simulink model "dmpwalk2014"  (R2018b)
settings: Solver=VariableStepAuto  StartTime=0.0  StopTime=100  RelTol=1e-3
values from neighbouring files (symbols this model uses):
  arm_radius = leg_radius    (= 0.01)    [Nao_paramter.m]
  foot_height = 0.02    [Nao_paramter.m]
  foot_length = 0.1    [Nao_paramter.m]
  foot_mass = 0.17184    [Nao_paramter.m]
  foot_width = 0.05    [Nao_paramter.m]
  ground_height = 0.0025    [Nao_paramter.m]
  ground_length = 5    [Nao_paramter.m]
  ground_width = 2    [Nao_paramter.m]
  hand_mass = 0.18533    [Nao_paramter.m]
  head_mass = 0.60533    [Nao_paramter.m]
  hip_mass = 0.14053    [Nao_paramter.m]
  hip_off_Y = 0.05    [Nao_paramter.m]
  hip_off_Z = 0.085    [Nao_paramter.m]
  leg_radius = 0.01    [Nao_paramter.m]
  lowerarm_length = 0.05595    [Nao_paramter.m]
  lowerarm_mass = 0.07761    [Nao_paramter.m]
  neck_length = 0.03    [Nao_paramter.m]
  neck_mass = 0.07842    [Nao_paramter.m]
  neck_off_Z = 0.1265    [Nao_paramter.m]
  shoulder_mass = 0.09304    [Nao_paramter.m]
  thigh_mass = 0.38968    [Nao_paramter.m]
  tibia_mass = 0.30142    [Nao_paramter.m]
  torso_height = foot_height + tibia_length + thigh_length + 0.5*hip_off_Z    (= 0.2654)    [Nao_paramter.m]
  torso_mass = 1.0496    [Nao_paramter.m]
  upperarm_length = 0.105    [Nao_paramter.m]
  upperarm_mass = 0.15777    [Nao_paramter.m]
undefined symbols (not defined in the file or in its folder): sigbuilder_block, X, Y, Z
libraries: sm_lib x87, nesl_utility x15, Contact_Forces_Lib x10
(part 4 of 5)

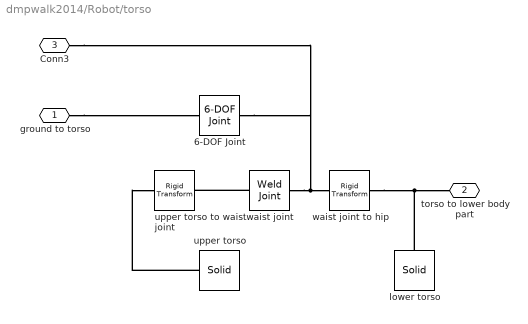
== system dmpwalk2014/Robot/torso ==
  " waist joint" : sm_lib/Joints/Weld Joint  SenseConstraintForce=off  SenseConstraintForceX=off  SenseConstraintForceY=off  SenseConstraintForceZ=off  SenseConstraintTorque=off  SenseConstraintTorqueX=off  SenseConstraintTorqueY=off  SenseConstraintTorqueZ=off  SenseTotalForce=off  SenseTotalForceX=off  SenseTotalForceY=off  SenseTotalForceZ=off  SenseTotalTorque=off  SenseTotalTorqueX=off  SenseTotalTorqueY=off  SenseTotalTorqueZ=off  CompositeWrenchDir=FollowerOnBase  CompositeWrenchFrame=BaseFrame
  6-DOF Joint : sm_lib/Joints/6-DOF Joint  SenseConstraintForce=off  SenseConstraintForceX=off  SenseConstraintForceY=off  SenseConstraintForceZ=off  SenseConstraintTorque=off  SenseConstraintTorqueX=off  SenseConstraintTorqueY=off  SenseConstraintTorqueZ=off  SenseTotalForce=off  SenseTotalForceX=off  SenseTotalForceY=off  SenseTotalForceZ=off  SenseTotalTorque=off  SenseTotalTorqueX=off  SenseTotalTorqueY=off  SenseTotalTorqueZ=off  CompositeWrenchDir=FollowerOnBase  CompositeWrenchFrame=BaseFrame  PxEquilibriumPosition=0  PxEquilibriumPositionUnits=m  PxSpringStiffness=1000  PxSpringStiffnessUnits=N/m  PxDampingCoefficient=800  PxDampingCoefficientUnits=N/(m/s)  PxTorqueActuationMode=NoTorque  PxMotionActuationMode=ComputedMotion  PxSensePosition=off  PxSenseVelocity=off  PxSenseAcceleration=off  PxSenseTorqueForce=off  PxPositionTargetSpecify=on  PxPositionTargetPriority=High  PxPositionTargetValue=0  PxPositionTargetValueUnits=m  PxVelocityTargetSpecify=off  PxVelocityTargetPriority=High  PxVelocityTargetValue=0  PxVelocityTargetValueUnits=m/s  PyEquilibriumPosition=0  PyEquilibriumPositionUnits=m  PySpringStiffness=1000  PySpringStiffnessUnits=N/m  PyDampingCoefficient=800  PyDampingCoefficientUnits=N/(m/s)  PyTorqueActuationMode=NoTorque  PyMotionActuationMode=ComputedMotion  PySensePosition=off  PySenseVelocity=off  PySenseAcceleration=off  PySenseTorqueForce=off  PyPositionTargetSpecify=on  PyPositionTargetPriority=High  PyPositionTargetValue=0  PyPositionTargetValueUnits=m  PyVelocityTargetSpecify=off  PyVelocityTargetPriority=High  PyVelocityTargetValue=0  PyVelocityTargetValueUnits=m/s  PzEquilibriumPosition=0  PzEquilibriumPositionUnits=m  PzSpringStiffness=1000  PzSpringStiffnessUnits=N/m  PzDampingCoefficient=800  PzDampingCoefficientUnits=N/(m/s)  PzTorqueActuationMode=NoTorque  PzMotionActuationMode=ComputedMotion  PzSensePosition=off  PzSenseVelocity=off  PzSenseAcceleration=off  PzSenseTorqueForce=off  PzPositionTargetSpecify=on  PzPositionTargetPriority=High  PzPositionTargetValue=torso_height+0.001  PzPositionTargetValueUnits=m  PzVelocityTargetSpecify=off  PzVelocityTargetPriority=High  PzVelocityTargetValue=0  PzVelocityTargetValueUnits=m/s  SphDefPosRotationMethod=None  SphDefPosRotationAngleUnits=deg  SphDefPosRotationStandardAxis=+Z  SphDefPosRotationAngle=0.0  SphDefPosRotationArbitraryAxis=[0 0 1]  SphDefPosFollAlignAxisA=+X  SphDefPosBaseAlignAxisA=+Y  SphDefPosFollAlignAxisB=+Y  SphDefPosBaseAlignAxisB=+Z  SphDefPosRotationSequenceAxes=FollowerAxes  SphDefPosRotationSequence=XYX  SphDefPosRotationSequenceAngles=[0 0 0]  SphDefPosRotationSequenceAnglesUnits=deg  SphDefPosRotationMatrix=[1 0 0; 0 1 0; 0 0 1]  SphEqPosRotationMethod=None  SphEqPosRotationAngleUnits=deg  SphEqPosRotationStandardAxis=+Z  SphEqPosRotationAngle=0.0  SphEqPosRotationArbitraryAxis=[0 0 1]  SphEqPosFollAlignAxisA=+X  SphEqPosBaseAlignAxisA=+Y  SphEqPosFollAlignAxisB=+Y  SphEqPosBaseAlignAxisB=+Z  SphEqPosRotationSequenceAxes=FollowerAxes  SphEqPosRotationSequence=XYX  SphEqPosRotationSequenceAngles=[0 0 0]  SphEqPosRotationSequenceAnglesUnits=deg  SphEqPosRotationMatrix=[1 0 0; 0 1 0; 0 0 1]  SphSpringStiffness=1000  SphSpringStiffnessUnits=N*m/deg  SphDampingCoefficient=1000  SphDampingCoefficientUnits=N*m/(rad/s)  SphActuateTorqueX=off  SphActuateTorqueY=off  SphActuateTorqueZ=off  SphActuateTorque=off  SphTorqueActuationMode=NoTorque  SphMotionActuationMode=ComputedMotion  SphActuationFrame=BaseFrame  SphSensePosition=off  SphSenseVelocityX=off  SphSenseVelocityY=off  SphSenseVelocityZ=off  SphSenseVelocity=off  SphSenseAccelerationX=off  SphSenseAccelerationY=off  SphSenseAccelerationZ=off  SphSenseAcceleration=off  SphSenseTorqueX=off  SphSenseTorqueY=off  SphSenseTorqueZ=off  SphSenseTorqueForce=off  SphSensingFrame=BaseFrame  SphPositionTargetRotationMethod=None  SphPositionTargetRotationAngleUnits=deg  SphPositionTargetRotationStandardAxis=+Z  SphPositionTargetRotationAngle=0.0  SphPositionTargetRotationArbitraryAxis=[0 0 1]  SphPositionTargetFollAlignAxisA=+X  SphPositionTargetBaseAlignAxisA=+Y  SphPositionTargetFollAlignAxisB=+Y  SphPositionTargetBaseAlignAxisB=+Z  SphPositionTargetRotationSequenceAxes=FollowerAxes  SphPositionTargetRotationSequence=XYX  SphPositionTargetRotationSequenceAngles=[0 0 0]  SphPositionTargetRotationSequenceAnglesUnits=deg  SphPositionTargetRotationMatrix=eye(3)  SphPositionTargetSpecify=off  SphPositionTargetPriority=High  SphVelocityTargetValue=[0 0 0]  SphVelocityTargetValueUnits=deg/s  SphVelocityTargetSpecify=off  SphVelocityTargetPriority=High  SphVelocityTargetInFollowerFrame=on
  lower torso : sm_lib/Body Elements/Solid  InertiaType=CalculateFromGeometry  Mass=hip_mass  MassUnits=kg  CenterOfMass=[0 0 0]  CenterOfMassUnits=m  MomentsOfInertia=[1 1 1]  MomentsOfInertiaUnits=kg*m^2  ProductsOfInertia=[1 1 1]  ProductsOfInertiaUnits=kg*m^2  BasedOnType=Mass  Density=1000  DensityUnits=kg/m^3  DoExposeReferenceFrame=on  SerializedFrames=<Frames/>  GraphicType=FromGeometry  MarkerShape=Sphere  MarkerSize=10  GraphicVisPropType=SimpleVisualProperties  GraphicDiffuseColor=[0.6 0.6 0.6]  GraphicSpecularColor=[0.5 0.5 0.5 1.0]  GraphicAmbientColor=[0.15 0.15 0.15 1.0]  GraphicEmissiveColor=[0.0 0.0 0.0 1.0]  GraphicShininess=75  GraphicOpacity=1.0  GeometryShape=Brick  RectangleSize=[1 1]  RectangleSizeUnits=m  BrickDimensions=[0.5*foot_length 2*hip_off_Y hip_off_Z]  BrickDimensionUnits=m  CylinderRadius=1  CylinderRadiusUnits=m  CylinderLength=1  CylinderLengthUnits=m  SphereRadius=1  SphereRadiusUnits=m  EllipsoidRadii=[1 1 1]  EllipsoidRadiiUnits=m  ExtrusionCrossSection=[1 1; -1 1; -1 -1; 1 -1]  ExtrusionCrossSectionUnits=m  ExtrusionLength=1  ExtrusionLengthUnits=m  PolygonNumSides=3  PolygonOuterRadius=1  PolygonOuterRadiusUnits=m  ExtGeomFileType=STEP  ExtGeomFileUnits=m  RevolutionCrossSection=[1 1; 1 -1; 2 -1; 2 1]  RevolutionCrossSectionUnits=m  RevolutionExtent=Full  RevolutionAngle=180  RevolutionAngleUnits=deg
  upper torso : sm_lib/Body Elements/Solid  InertiaType=Custom  Mass=torso_mass  MassUnits=kg  CenterOfMass=[-0.00413 0 0.5*neck_off_Z]  CenterOfMassUnits=m  MomentsOfInertia=torso_inertia_m  MomentsOfInertiaUnits=kg*m^2  ProductsOfInertia=torso_inertia_p  ProductsOfInertiaUnits=kg*m^2  BasedOnType=Mass  Density=1000  DensityUnits=kg/m^3  DoExposeReferenceFrame=on  SerializedFrames=<Frames/>  GraphicType=FromGeometry  MarkerShape=Sphere  MarkerSize=10  GraphicVisPropType=SimpleVisualProperties  GraphicDiffuseColor=[0.5 0.5 0.5]  GraphicSpecularColor=[0.5 0.5 0.5 1.0]  GraphicAmbientColor=[0.15 0.15 0.15 1.0]  GraphicEmissiveColor=[0.0 0.0 0.0 1.0]  GraphicShininess=75  GraphicOpacity=1.0  GeometryShape=Brick  RectangleSize=[1 1]  RectangleSizeUnits=m  BrickDimensions=[2*hip_off_Y 2.5*foot_width neck_off_Z]  BrickDimensionUnits=m  CylinderRadius=1  CylinderRadiusUnits=m  CylinderLength=1  CylinderLengthUnits=m  SphereRadius=1  SphereRadiusUnits=m  EllipsoidRadii=[1 1 1]  EllipsoidRadiiUnits=m  ExtrusionCrossSection=[1 1; -1 1; -1 -1; 1 -1]  ExtrusionCrossSectionUnits=m  ExtrusionLength=1  ExtrusionLengthUnits=m  PolygonNumSides=3  PolygonOuterRadius=1  PolygonOuterRadiusUnits=m  ExtGeomFileType=STEP  ExtGeomFileUnits=m  RevolutionCrossSection=[1 1; 1 -1; 2 -1; 2 1]  RevolutionCrossSectionUnits=m  RevolutionExtent=Full  RevolutionAngle=180  RevolutionAngleUnits=deg
  upper torso to waist joint : sm_lib/Frames and Transforms/Rigid Transform  TranslationMethod=StandardAxis  TranslationStandardOffset=0.5*neck_off_Z  TranslationLengthUnit=m  TranslationStandardAxis=-Z  TranslationCartesianOffset=[0 0 0]  TranslationROffset=0  TranslationROffsetUnits=m  TranslationZOffset=0  TranslationZOffsetUnits=m  TranslationThetaOffset=0  TranslationThetaOffsetUnits=deg  RotationMethod=None  RotationAngleUnits=deg  RotationStandardAxis=+Z  RotationAngle=0.0  RotationArbitraryAxis=[0 0 1]  FollAlignAxisA=+X  BaseAlignAxisA=+Y  FollAlignAxisB=+Y  BaseAlignAxisB=+Z  RotationSequenceAxes=FollowerAxes  RotationSequence=XYX  RotationSequenceAngles=[0 0 0]  RotationSequenceAnglesUnits=deg  RotationMatrix=[1 0 0; 0 1 0; 0 0 1]
  waist joint to hip : sm_lib/Frames and Transforms/Rigid Transform  TranslationMethod=StandardAxis  TranslationStandardOffset=0.5*hip_off_Z  TranslationLengthUnit=m  TranslationStandardAxis=-Z  TranslationCartesianOffset=[0 0 0]  TranslationROffset=0  TranslationROffsetUnits=m  TranslationZOffset=0  TranslationZOffsetUnits=m  TranslationThetaOffset=0  TranslationThetaOffsetUnits=deg  RotationMethod=None  RotationAngleUnits=deg  RotationStandardAxis=+Z  RotationAngle=0.0  RotationArbitraryAxis=[0 0 1]  FollAlignAxisA=+X  BaseAlignAxisA=+Y  FollAlignAxisB=+Y  BaseAlignAxisB=+Z  RotationSequenceAxes=FollowerAxes  RotationSequence=XYX  RotationSequenceAngles=[0 0 0]  RotationSequenceAnglesUnits=deg  RotationMatrix=[1 0 0; 0 1 0; 0 0 1]
  ground to torso : PMIOPort  Side=Left
  torso to lower body part : PMIOPort  Port=2  Side=Right
  Conn3 : PMIOPort  Port=3  Side=Left
  connections:
  upper torso/RConn1 -- upper torso to waist joint/LConn1
  " waist joint"/RConn1 -- 6-DOF Joint/RConn1 -- Conn3/RConn1 -- waist joint to hip/LConn1
  waist joint to hip/RConn1 -- lower torso/RConn1 -- torso to lower body part/RConn1
  " waist joint"/LConn1 -- upper torso to waist joint/RConn1
  ground to torso/RConn1 -- 6-DOF Joint/LConn1

== stateflow chart dmpwalk2014/motion planning1 ==
  state startStep
    entry:
    tau = 1;
    sDStart = tau*1.35;
    kStartMax = sDStart*100+1;
    [hPil,hPir,kBel,kBer,aPil,aPir,hRol,hRor,aRol,aRor,hYal,hYar] = motionStart(tau);
    state outStart
      entry:
      k = k+1;
      hipRollR = hRor(k);
      hipRollL = hRol(k);
      hipPitchR = hPir(k);
      hipPitchL = hPil(k);
      hipYawR = hYar(k);
      hipYawL = hYal(k);
      kneeBendR = kBer(k);
      kneeBendL = kBel(k);
      ankleRollR = aRor(k);
      ankleRollL = aRol(k);
      anklePitchR = aPir(k);
      anklePitchL = aPil(k);
    (default) -> outStart : {k=0;}
    outStart -> outStart : after(0.01,sec)
  state footRecover1
    entry:
    timeRecover = 0.1;
    footPos = [hPil(k),hPir(k),kBel(k),kBer(k),aPil(k),aPir(k),hRol(k),hRor(k),aRol(k),aRor(k),hYal(k),hYar(k)]
    [hPil,hPir,kBel,kBer,aPil,aPir,hRol,hRor,aRol,aRor,hYal,hYar] = footPosRecover(footPos,timeRecover);
    state outRecover
      entry:
      k = k+1;
      hipRollR = hRor(k);
      hipRollL = hRol(k);
      hipPitchR = hPir(k);
      hipPitchL = hPil(k);
      hipYawR = hYar(k);
      hipYawL = hYal(k);
      kneeBendR = kBer(k);
      kneeBendL = kBel(k);
      ankleRollR = aRor(k);
      ankleRollL = aRol(k);
      anklePitchR = aPir(k);
      anklePitchL = aPil(k);
    (default) -> footRecover1.outRecover : {k=0;}
    footRecover1.outRecover -> footRecover1.outRecover : after(0.01,sec)
  state stepStraightLeft
    entry:
    sDStrL = tau*1.05 ;
    kStrLMax = sDStrL*100+1
    [hPil,hPir,kBel,kBer,aPil,aPir,hRol,hRor,aRol,aRor,hYal,hYar] = motionStrWL(tau,countStrWL);
    state outStrL
      entry:
      k = k+1;
      hipRollR = hRor(k);
      hipRollL = hRol(k);
      hipPitchR = hPir(k);
      hipPitchL = hPil(k);
      hipYawR = hYar(k);
      hipYawL = hYal(k);
      kneeBendR = kBer(k);
      kneeBendL = kBel(k);
      ankleRollR = aRor(k);
      ankleRollL = aRol(k);
      anklePitchR = aPir(k);
      anklePitchL = aPil(k);
    (default) -> outStrL : {k=0;}
    outStrL -> outStrL : after(0.01,sec)
  state stepStraightRight
    entry:
    sDStrR = tau*1.10 ;
    kStrRMax = sDStrR*100+1
    [hPil,hPir,kBel,kBer,aPil,aPir,hRol,hRor,aRol,aRor,hYal,hYar] = motionStrWR(tau,countStrWR);
    state outStrR
      entry:
      k = k+1;
      hipRollR = hRor(k);
      hipRollL = hRol(k);
      hipPitchR = hPir(k);
      hipPitchL = hPil(k);
      hipYawR = hYar(k);
      hipYawL = hYal(k);
      kneeBendR = kBer(k);
      kneeBendL = kBel(k);
      ankleRollR = aRor(k);
      ankleRollL = aRol(k);
      anklePitchR = aPir(k);
      anklePitchL = aPil(k);
    (default) -> outStrR : {k=0;}
    outStrR -> outStrR : after(0.01,sec)
  state footRecover
    entry:
    timeRecover = 0.1;
    footPos = [hPil(k),hPir(k),kBel(k),kBer(k),aPil(k),aPir(k),hRol(k),hRor(k),aRol(k),aRor(k),hYal(k),hYar(k)]
    [hPil,hPir,kBel,kBer,aPil,aPir,hRol,hRor,aRol,aRor,hYal,hYar] = footPosRecover(footPos,timeRecover);
    state outRecover
      entry:
      k = k+1;
      hipRollR = hRor(k);
      hipRollL = hRol(k);
      hipPitchR = hPir(k);
      hipPitchL = hPil(k);
      hipYawR = hYar(k);
      hipYawL = hYal(k);
      kneeBendR = kBer(k);
      kneeBendL = kBel(k);
      ankleRollR = aRor(k);
      ankleRollL = aRol(k);
      anklePitchR = aPir(k);
      anklePitchL = aPil(k);
    (default) -> footRecover.outRecover : {k=0;}
    footRecover.outRecover -> footRecover.outRecover : after(0.01,sec)
  state stepEnd
    entry:
    sDEnd = tau*2 ;
    kEndMax = sDEnd*100+1
    [hPil,hPir,kBel,kBer,aPil,aPir,hRol,hRor,aRol,aRor,hYal,hYar] = motionEndstep(tau);
    state outEnd
      entry:
      k = k+1;
      hipRollR = hRor(k);
      hipRollL = hRol(k);
      hipPitchR = hPir(k);
      hipPitchL = hPil(k);
      hipYawR = hYar(k);
      hipYawL = hYal(k);
      kneeBendR = kBer(k);
      kneeBendL = kBel(k);
      ankleRollR = aRor(k);
      ankleRollL = aRol(k);
      anklePitchR = aPir(k);
      anklePitchL = aPil(k);
    (default) -> outEnd : {k=0;}
    outEnd -> outEnd : after(0.01,sec)
  state stepSideRight
    entry:
    sDSideR = tau*1.63 ;
    kSideR = sDSideR*100+1
    [hPil,hPir,kBel,kBer,aPil,aPir,hRol,hRor,aRol,aRor,hYal,hYar] = motionSideRight(tau,countSideR);
    state outSideR
      entry:
      k = k+1;
      hipRollR = hRor(k);
      hipRollL = hRol(k);
      hipPitchR = hPir(k);
      hipPitchL = hPil(k);
      hipYawR = hYar(k);
      hipYawL = hYal(k);
      kneeBendR = kBer(k);
      kneeBendL = kBel(k);
      ankleRollR = aRor(k);
      ankleRollL = aRol(k);
      anklePitchR = aPir(k);
      anklePitchL = aPil(k);
    (default) -> outSideR : {k=0;}
    outSideR -> outSideR : after(0.01,sec)
  state stepSideLeft
    entry:
    sDSideL = tau*0.75;
    kSideL = sDSideL*100+1
    [hPil,hPir,kBel,kBer,aPil,aPir,hRol,hRor,aRol,aRor,hYal,hYar] = motionSideLeft(tau);
    state outSideL
      entry:
      k = k+1;
      hipRollR = hRor(k);
      hipRollL = hRol(k);
      hipPitchR = hPir(k);
      hipPitchL = hPil(k);
      hipYawR = hYar(k);
      hipYawL = hYal(k);
      kneeBendR = kBer(k);
      kneeBendL = kBel(k);
      ankleRollR = aRor(k);
      ankleRollL = aRol(k);
      anklePitchR = aPir(k);
      anklePitchL = aPil(k);
    (default) -> outSideL : {k=0;}
    outSideL -> outSideL : after(0.01,sec)
  state kick
    entry:
    sDKick = tau*2.78;
    kKick = sDKick*100+1
    [hPil,hPir,kBel,kBer,aPil,aPir,hRol,hRor,aRol,aRor,hYal,hYar] = motionKick(tau);
    state outKick
      entry:
      k = k+1;
      hipRollR = hRor(k);
      hipRollL = hRol(k);
      hipPitchR = hPir(k);
      hipPitchL = hPil(k);
      hipYawR = hYar(k);
      hipYawL = hYal(k);
      kneeBendR = kBer(k);
      kneeBendL = kBel(k);
      ankleRollR = aRor(k);
      ankleRollL = aRol(k);
      anklePitchR = aPir(k);
      anklePitchL = aPil(k);
    (default) -> outKick : {k=0;}
    outKick -> outKick : after(0.01,sec)
  state stop1 [commented out]
    entry:
    stop = 1;
    stopWalking(stop);
    state stopWalking(in) [function] [commented out]
  (default) -> startStep
  footRecover1 -> stepStraightLeft : after(timeRecover,sec)
  startStep -> stepStraightLeft : after(sDStart,sec)[rp > 200]{nStraight = 10; countStrWL = 0; countStrWR = 0;}
  (junction 1184) -> footRecover1 [order 2] : [rp < 200]
  (junction 1184) -> stepStraightLeft [order 1] : [rp > 200]
  stepStraightRight -> (junction 1184) : after(sDStrR,sec){countStrWR = countStrWR+1;}
  stepStraightLeft -> (junction 1043) : after(sDStrL,sec)[lp > 200]{countStrWL = countStrWL+1;}
  (junction 1043) -> stepStraightRight [order 1] : [countStrWL < 10]
  footRecover -> stepSideLeft : after(timeRecover,sec)
  (junction 1043) -> stepEnd [order 2] : [countStrWL >= 10]
  (junction 1139) -> footRecover [order 2] : [rp <= 10]
  stepSideRight -> (junction 1139) : after(sDSideR,sec){countSideR = countSideR+1;}
  (junction 1139) -> stepSideLeft [order 1] : [rp > 10]
  stepEnd -> stepSideRight : after(sDEnd,sec)[lp > 200]{countSideL = 0;countSideR = 0;}
  (junction 1110) -> stepSideRight [order 1] : [countSideL < 20]
  stepSideLeft -> (junction 1110) : after(sDSideL,sec)[lp > 10]{countSideL = countSideL+1;}
  (junction 1110) -> kick [order 2] : [countSideL >= 20]
  kick -> stop1 [commented out] : after(sDKick,sec)
  data: hPl function_output; hPr function_output; kBl function_output; kBr function_output; aPl function_output; aPr function_output; hRl function_output; tScale function_input; hRr function_output; aRl function_output; aRr function_output; hYl function_output; hYr function_output; hPlRe function_output; hPrRe function_output; kBlRe function_output; kBrRe function_output; aPlRe function_output; aPrRe function_output; hRlRe function_output; pos function_input; tR function_input; hRrRe function_output; aRlRe function_output; aRrRe function_output; hYlRe function_output; hYrRe function_output; hPl function_output; hPr function_output; kBl function_output; kBr function_output; aPl function_output; aPr function_output; hRl function_output; tScale function_input; count function_input; hRr function_output; aRl function_output; aRr function_output; hYl function_output; hYr function_output; hPl function_output; hPr function_output; kBl function_output; kBr function_output; aPl function_output; aPr function_output; hRl function_output; tScale function_input; count function_input; hRr function_output; aRl function_output; aRr function_output; hYl function_output; hYr function_output; hPlRe function_output; hPrRe function_output; kBlRe function_output; kBrRe function_output; aPlRe function_output; aPrRe function_output; hRlRe function_output; pos function_input; tR function_input; hRrRe function_output; aRlRe function_output; aRrRe function_output; hYlRe function_output; hYrRe function_output; hPl function_output; hPr function_output; kBl function_output; kBr function_output; aPl function_output; aPr function_output; hRl function_output; tScale function_input; count function_input; hRr function_output; aRl function_output; aRr function_output; hYl function_output; hYr function_output; hPl function_output; hPr function_output; kBl function_output; kBr function_output; aPl function_output; aPr function_output; hRl function_output; tScale function_input; count function_input; hRr function_output; aRl function_output; aRr function_output; hYl function_output; hYr function_output; hPl function_output; hPr function_output; kBl function_output; kBr function_output; aPl function_output; aPr function_output; hRl function_output; tScale function_input; count function_input; hRr function_output; aRl function_output; aRr function_output; hYl function_output; hYr function_output; hPl function_output; hPr function_output; kBl function_output; kBr function_output; aPl function_output; aPr function_output; hRl function_output; tScale function_input; hRr function_output; aRl function_output; aRr function_output; hYl function_output; hYr function_output; in function_input double size=1; hipRollL output; hipRollR output; hipPitchL output; hipPitchR output; hipYawL output; hipYawR output; kneeBendL output; kneeBendR output; rp input; lp input; k local; ankleRollL output; ankleRollR output; anklePitchL output; anklePitchR output; aPil local size=[1 2000]; aPir local size=[1 2000]; aRol local size=[1 2000]; aRor local size=[1 2000]; hPil local size=[1 2000]; hPir local size=[1 2000]; hRol local size=[1 2000]; hRor local size=[1 2000]; hYal local size=[1 2000]; hYar local size=[1 2000]; kBel local size=[1 2000]; kBer local size=[1 2000]; tau local; sDStart local; kStartMax local; nStraight local; motionStartFinal local; countSide local; motionSideFinal local double size=[10 1]; nSide local; countEnd local; kEndMax local; motionEndFinal local; nEnd local; sDEnd local; stop local; sDKick local; nKick local; motionKickFinal local; kKickMax local; countKick local; LR local; kSideLMax local; kSideRMax local; sDSideL local; sDSideR local; countStraight local; motionStraighFinal local; sDStraight local; kStraightMax local; motionStraightFinal local; mtionKickFinal local; kStrRMax local; sDStrR local; motionStrWLFinalFinal local; motionStrWLFinal local; kStrLMax local; sDStrL local; motionStrWRFinal local; countStrWL local; countStrWR local; kKick local; kSideL local; kSideR local; countSideL local; countSideR local; footPos local; timeRecover local
  function [hPl,hPr,kBl,kBr,aPl,aPr,hRl,hRr,aRl,aRr,hYl,hYr] = motionStart(tScale):
    | function [hPl,hPr,kBl,kBr,aPl,aPr,hRl,hRr,aRl,aRr,hYl,hYr] = motionStart(tScale)
    | 
    | 
    | w = load ('wBegstep.mat');
    | p = load ('primiBegstep.mat');
    | 
    | dt = 0.01;
    | N_dmp = 10;     % number of dmps, number of curves to be imitated 
    | N_bf = 50;     % number of basic activation function
    | weights = zeros(N_dmp,N_bf);
    | ay = 25;        % ay & by: constants of the second order system
    | by = ay/4;
    | t = 0:dt:dt*(size(p.primiBegstep,2)-1);
    | t1 = 0:dt:tScale*t(end); 
    | anglesIm1 = zeros(10,length(t1));
    | ax = 1;
    | %%
    | for j = 1:N_dmp
    |     
    |     y0 = p.primiBegstep(j,1);
    |     yg = p.primiBegstep(j,end);
    |     x1 = exp(-ax/tScale*t1);
    |     des_c1 = linspace(0,max(t1),N_bf);    % point in time where to put the activation function
    |     c1 = exp(-ax/tScale*des_c1);             % point in x where to put the activation function
    |     h1 = N_bf^1.5*ones(1,N_bf)./c1;       % variance of each activation function, trial and error
    | 
    |     psi1 = zeros(N_bf,length(x1));
    |         for k = 1:N_bf
    |             for l = 1:length(x1)
    |                 psi1(k,l) = exp(-h1(k)*(x1(l)-c1(k))^2);
    |             end
    |         end    
    |         
    |     % Forcing term
    |     wpsi1 = w.wBegstep(j,:)*psi1;
    |     f1 = wpsi1./(sum(psi1)).*x1*(yg-y0);
    |     
    |     % Reproducing
    |     ddyIm = zeros(1,length(t1));
    |     dyIm = zeros(1,length(t1));
    |     yIm = zeros(1,length(t1));
    |     yIm(1) = y0;
    |     
    |     for k = 2:length(t1)
    |         ddyIm(k-1) = 1/tScale^2*(ay*(by*(yg-yIm(k-1))-tScale*dyIm(k-1))+f1(k-1));
    |         dyIm(k) = dyIm(k-1)+ddyIm(k-1)*dt;
    |         yIm(k) = yIm(k-1)+dyIm(k-1)*dt;
    |     end
    |     
    |     anglesIm1(j,:) = yIm;
    | end
    | 
    | 
    | 
    | 
    | 
    | hPl = anglesIm1(1,:);
    | hPr = anglesIm1(2,:);
    | kBl = anglesIm1(3,:);
    | kBr = anglesIm1(4,:);
    | aPl = anglesIm1(5,:);
    | aPr = anglesIm1(6,:);
    | hRl = -anglesIm1(7,:);
    | hRr = -anglesIm1(8,:);
    | aRl = -anglesIm1(9,:);
    | aRr = -anglesIm1(10,:);
    | hYl = zeros(1,size(anglesIm1,2));   
    | hYr = zeros(1,size(anglesIm1,2));
  function [hPlRe,hPrRe,kBlRe,kBrRe,aPlRe,aPrRe,hRlRe,hRrRe,aRlRe,aRrRe,hYlRe,hYrRe] = footPosRecover(pos,tR):
    | function [hPlRe,hPrRe,kBlRe,kBrRe,aPlRe,aPrRe,hRlRe,hRrRe,aRlRe,aRrRe,hYlRe,hYrRe] = footPosRecover(pos,tR)
    | 
    | pos = pos';
    | pR = load('primiRightstep');
    | des = pR.primiRightstep(:,end);
    | des(7:10,:) = -des(7:10,:);
    | re = pchip([0,tR],[pos(1:10,:),des],0:0.01:tR);
    | % re = pchip([0,tR],[zeros(10,1),des],0:0.01:tR);
    | hPlRe = re(1,:);
    | hPrRe = re(2,:);
    | kBlRe = re(3,:);
    | kBrRe = re(4,:);
    | aPlRe = -hPlRe+kBlRe;%anglesIm1(5,:);
    | aPrRe = -hPrRe+kBrRe;%anglesIm1(6,:);
    | hRlRe = re(7,:);
    | hRrRe = re(8,:);
    | aRlRe = re(9,:);
    | aRrRe = re(10,:);
    | hYlRe = zeros(1,size(re,2));   
    | hYrRe = zeros(1,size(re,2));
    | 
    | % hPlRe = pos(1,:)+re(1,:);
    | % hPrRe = pos(2,:)+re(2,:);
    | % kBlRe = pos(3,:)+re(3,:);
    | % kBrRe = pos(4,:)+re(4,:);
    | % aPlRe = -hPlRe+kBlRe;%anglesIm1(5,:);
    | % aPrRe = -hPrRe+kBrRe;%anglesIm1(6,:);
    | % hRlRe = pos(7,:)-re(7,:);
    | % hRrRe = pos(8,:)-re(8,:);
    | % aRlRe = pos(9,:)-re(9,:);
    | % aRrRe = pos(10,:)-re(10,:);
    | % hYlRe = zeros(1,size(re,2));   
    | % hYrRe = zeros(1,size(re,2));
  function [hPl,hPr,kBl,kBr,aPl,aPr,hRl,hRr,aRl,aRr,hYl,hYr] = motionStrWL(tScale,count):
    | function [hPl,hPr,kBl,kBr,aPl,aPr,hRl,hRr,aRl,aRr,hYl,hYr] = motionStrWL(tScale,count)
    | 
    | 
    | w = load ('wLeftstep.mat');
    | pStart = load ('primiBegstep.mat');
    | pL = load ('primiLeftstep.mat');
    | pR = load ('primiRightstep.mat');
    | 
    | dt = 0.01;
    | N_dmp = 10;     % number of dmps, number of curves to be imitated 
    | N_bf = 50;     % number of basic activation function
    | weights = zeros(N_dmp,N_bf);
    | ay = 25;        % ay & by: constants of the second order system
    | by = ay/4;
    | t = 0:dt:dt*(size(pL.primiLeftstep,2)-1);
    | t1 = 0:dt:tScale*t(end);
    | anglesIm1 = zeros(10,length(t1));
    | ax = 1;
    | %%
    | for j = 1:N_dmp
    |     
    |     y0 = pL.primiLeftstep(j,1);
    |     yg = pL.primiLeftstep(j,end);
    |     x1 = exp(-ax/tScale*t1);
    |     des_c1 = linspace(0,max(t1),N_bf);    % point in time where to put the activation function
    |     c1 = exp(-ax/tScale*des_c1);             % point in x where to put the activation function
    |     h1 = N_bf^1.5*ones(1,N_bf)./c1;       % variance of each activation function, trial and error
    | 
    |     psi1 = zeros(N_bf,length(x1));
    |         for k = 1:N_bf
    |             for l = 1:length(x1)
    |                 psi1(k,l) = exp(-h1(k)*(x1(l)-c1(k))^2);
    |             end
    |         end    
    |         
    |     % Forcing term
    |     wpsi1 = w.wLeftstep(j,:)*psi1;
    |     f1 = wpsi1./(sum(psi1)).*x1*(yg-y0);
    |     
    |     % Reproducing
    |     ddyIm = zeros(1,length(t1));
    |     dyIm = zeros(1,length(t1));
    |     yIm = zeros(1,length(t1));
    |     
    |     if count == 1
    |         yIm(1) = pStart.primiBegstep(j,end);
    |     else
    |         yIm(1) = pR.primiRightstep(j,end);
    |     end
    | 
    |     
    |     
    |     for k = 2:length(t1)
    |         ddyIm(k-1) = 1/tScale^2*(ay*(by*(yg-yIm(k-1))-tScale*dyIm(k-1))+f1(k-1));
    |         dyIm(k) = dyIm(k-1)+ddyIm(k-1)*dt;
    |         yIm(k) = yIm(k-1)+dyIm(k-1)*dt;  
    |     end
    |     
    |     anglesIm1(j,:) = yIm;
    | end
    | 
    | 
    | hPl = anglesIm1(1,:);
    | hPr = anglesIm1(2,:);
    | kBl = anglesIm1(3,:);
    | kBr = anglesIm1(4,:);
    | aPl = -hPl+kBl;%anglesIm1(5,:);
    | aPr = -hPr+kBr;%anglesIm1(6,:);
    | hRl = -anglesIm1(7,:);
    | hRr = -anglesIm1(8,:);
    | aRl = -anglesIm1(9,:);
    | aRr = -anglesIm1(10,:);
    | hYl = zeros(1,size(anglesIm1,2));   
    | hYr = zeros(1,size(anglesIm1,2));
  function [hPl,hPr,kBl,kBr,aPl,aPr,hRl,hRr,aRl,aRr,hYl,hYr] = motionStrWR(tScale,count):
    | function [hPl,hPr,kBl,kBr,aPl,aPr,hRl,hRr,aRl,aRr,hYl,hYr] = motionStrWR(tScale,count)
    | 
    | 
    | w = load ('wRightstep.mat');
    | pStart = load ('primiBegstep.mat');
    | pL = load ('primiLeftstep.mat');
    | pR = load ('primiRightstep.mat');
    | 
    | dt = 0.01;
    | N_dmp = 10;     % number of dmps, number of curves to be imitated 
    | N_bf = 50;     % number of basic activation function
    | weights = zeros(N_dmp,N_bf);
    | ay = 25;        % ay & by: constants of the second order system
    | by = ay/4;
    | t = 0:dt:dt*(size(pR.primiRightstep,2)-1);
    | t1 = 0:dt:tScale*t(end);
    | anglesIm1 = zeros(10,length(t1));
    | ax = 1;
    | %%
    | for j = 1:N_dmp
    |     
    |     y0 = pR.primiRightstep(j,1);
    |     yg = pR.primiRightstep(j,end);
    |     x1 = exp(-ax/tScale*t1);
    |     des_c1 = linspace(0,max(t1),N_bf);    % point in time where to put the activation function
    |     c1 = exp(-ax/tScale*des_c1);             % point in x where to put the activation function
    |     h1 = N_bf^1.5*ones(1,N_bf)./c1;       % variance of each activation function, trial and error
    | 
    |     psi1 = zeros(N_bf,length(x1));
    |         for k = 1:N_bf
    |             for l = 1:length(x1)
    |                 psi1(k,l) = exp(-h1(k)*(x1(l)-c1(k))^2);
    |             end
    |         end    
    |         
    |     % Forcing term
    |     wpsi1 = w.wRightstep(j,:)*psi1;
    |     f1 = wpsi1./(sum(psi1)).*x1*(yg-y0);
    |     
    |     % Reproducing
    |     ddyIm = zeros(1,length(t1));
    |     dyIm = zeros(1,length(t1));
    |     yIm = zeros(1,length(t1));
    |     
    | %     if count == 1
    |         yIm(1) = pL.primiLeftstep(j,end);
    | %     else
    | %         yIm(1) = ygEnd(j,1);
    | %     end
    | 
    |     
    |     
    |     for k = 2:length(t1)
    |         ddyIm(k-1) = 1/tScale^2*(ay*(by*(yg-yIm(k-1))-tScale*dyIm(k-1))+f1(k-1));
    |         dyIm(k) = dyIm(k-1)+ddyIm(k-1)*dt;
    |         yIm(k) = yIm(k-1)+dyIm(k-1)*dt;  
    |     end
    |     
    |     anglesIm1(j,:) = yIm;
    | end
    | 
    | 
    | hPl = anglesIm1(1,:);
    | hPr = anglesIm1(2,:);
    | kBl = anglesIm1(3,:);
    | kBr = anglesIm1(4,:);
    | aPl = -hPl+kBl;%anglesIm1(5,:);
    | aPr = -hPr+kBr;%anglesIm1(6,:);
    | hRl = -anglesIm1(7,:);
    | hRr = -anglesIm1(8,:);
    | aRl = -anglesIm1(9,:);
    | aRr = -anglesIm1(10,:);
    | hYl = zeros(1,size(anglesIm1,2));   
    | hYr = zeros(1,size(anglesIm1,2));
  function [hPlRe,hPrRe,kBlRe,kBrRe,aPlRe,aPrRe,hRlRe,hRrRe,aRlRe,aRrRe,hYlRe,hYrRe] = footPosRecover(pos,tR):
    | function [hPlRe,hPrRe,kBlRe,kBrRe,aPlRe,aPrRe,hRlRe,hRrRe,aRlRe,aRrRe,hYlRe,hYrRe] = footPosRecover(pos,tR)
    | 
    | pos = pos';
    | pSideR = load('primiRightside');
    | des = pSideR.primiRightside(:,end);
    | des(7:10,:) = -des(7:10,:);
    | re = pchip([0,tR],[pos(1:10,:),des],0:0.01:tR);
    | % re = pchip([0,tR],[zeros(10,1),des],0:0.01:tR);
    | hPlRe = re(1,:);
    | hPrRe = re(2,:);
    | kBlRe = re(3,:);
    | kBrRe = re(4,:);
    | aPlRe = -hPlRe+kBlRe;%anglesIm1(5,:);
    | aPrRe = -hPrRe+kBrRe;%anglesIm1(6,:);
    | hRlRe = re(7,:);
    | hRrRe = re(8,:);
    | aRlRe = re(9,:);
    | aRrRe = re(10,:);
    | hYlRe = zeros(1,size(re,2));   
    | hYrRe = zeros(1,size(re,2));
    | 
    | % hPlRe = pos(1,:)+re(1,:);
    | % hPrRe = pos(2,:)+re(2,:);
    | % kBlRe = pos(3,:)+re(3,:);
    | % kBrRe = pos(4,:)+re(4,:);
    | % aPlRe = -hPlRe+kBlRe;%anglesIm1(5,:);
    | % aPrRe = -hPrRe+kBrRe;%anglesIm1(6,:);
    | % hRlRe = pos(7,:)-re(7,:);
    | % hRrRe = pos(8,:)-re(8,:);
    | % aRlRe = pos(9,:)-re(9,:);
    | % aRrRe = pos(10,:)-re(10,:);
    | % hYlRe = zeros(1,size(re,2));   
    | % hYrRe = zeros(1,size(re,2));
  function [hPl,hPr,kBl,kBr,aPl,aPr,hRl,hRr,aRl,aRr,hYl,hYr] = motionEndstep(tScale,count):
    | function [hPl,hPr,kBl,kBr,aPl,aPr,hRl,hRr,aRl,aRr,hYl,hYr] = motionEndstep(tScale,count)
    | 
    | 
    | w = load ('wEndstep.mat');
    | pEnd = load ('primiEndstep.mat');
    | pL = load ('primiLeftstep.mat');
    | pR = load ('primiRightstep.mat');
    | 
    | dt = 0.01;
    | N_dmp = 10;     % number of dmps, number of curves to be imitated 
    | N_bf = 50;     % number of basic activation function
    | weights = zeros(N_dmp,N_bf);
    | ay = 25;        % ay & by: constants of the second order system
    | by = ay/4;
    | t = 0:dt:dt*(size(pEnd.primiEndstep,2)-1);
    | t1 = 0:dt:tScale*t(end);
    | anglesIm1 = zeros(10,length(t1));
    | ax = 1;
    | %%
    | for j = 1:N_dmp
    |     
    |     y0 = pEnd.primiEndstep(j,1);
    |     yg = pEnd.primiEndstep(j,end);
    |     x1 = exp(-ax/tScale*t1);
    |     des_c1 = linspace(0,max(t1),N_bf);    % point in time where to put the activation function
    |     c1 = exp(-ax/tScale*des_c1);             % point in x where to put the activation function
    |     h1 = N_bf^1.5*ones(1,N_bf)./c1;       % variance of each activation function, trial and error
    | 
    |     psi1 = zeros(N_bf,length(x1));
    |         for k = 1:N_bf
    |             for l = 1:length(x1)
    |                 psi1(k,l) = exp(-h1(k)*(x1(l)-c1(k))^2);
    |             end
    |         end    
    |         
    |     % Forcing term
    |     wpsi1 = w.wEndstep(j,:)*psi1;
    |     f1 = wpsi1./(sum(psi1)).*x1*(yg-y0);
    |     
    |     % Reproducing
    |     ddyIm = zeros(1,length(t1));
    |     dyIm = zeros(1,length(t1));
    |     yIm = zeros(1,length(t1));
    |     
    | %     if count == 1
    | %         yIm(1) = pEnd.primiBegstep(j,end);
    | %     else
    |         yIm(1) = pL.primiLeftstep(j,end);
    | %     end
    | 
    |     
    |     
    |     for k = 2:length(t1)
    |         ddyIm(k-1) = 1/tScale^2*(ay*(by*(yg-yIm(k-1))-tScale*dyIm(k-1))+f1(k-1));
    |         dyIm(k) = dyIm(k-1)+ddyIm(k-1)*dt;
    |         yIm(k) = yIm(k-1)+dyIm(k-1)*dt;  
    |     end
    |     
    |     anglesIm1(j,:) = yIm;
    | end
    | 
    | 
    | hPl = anglesIm1(1,:);
    | hPr = anglesIm1(2,:);
    | kBl = anglesIm1(3,:);
    | kBr = anglesIm1(4,:);
    | aPl = -hPl+kBl;%anglesIm1(5,:);
    | aPr = -hPr+kBr;%anglesIm1(6,:);
    | hRl = -anglesIm1(7,:);
    | hRr = -anglesIm1(8,:);
    | aRl = -anglesIm1(9,:);
    | aRr = -anglesIm1(10,:);
    | hYl = zeros(1,size(anglesIm1,2));   
    | hYr = zeros(1,size(anglesIm1,2));
  function [hPl,hPr,kBl,kBr,aPl,aPr,hRl,hRr,aRl,aRr,hYl,hYr] = motionSideRight(tScale,count):
    | function [hPl,hPr,kBl,kBr,aPl,aPr,hRl,hRr,aRl,aRr,hYl,hYr] = motionSideRight(tScale,count)
    | 
    | 
    | w = load ('wRightside.mat');
    | pEnd = load ('primiEndstep.mat');
    | pL = load ('primiLeftside.mat');
    | pR = load ('primiRightside.mat');
    | 
    | dt = 0.01;
    | N_dmp = 10;     % number of dmps, number of curves to be imitated 
    | N_bf = 50;     % number of basic activation function
    | weights = zeros(N_dmp,N_bf);
    | ay = 25;        % ay & by: constants of the second order system
    | by = ay/4;
    | t = 0:dt:dt*(size(pR.primiRightside,2)-1);
    | t1 = 0:dt:tScale*t(end);
    | anglesIm1 = zeros(10,length(t1));
    | ax = 1;
    | %%
    | for j = 1:N_dmp
    |     
    |     y0 = pR.primiRightside(j,1);
    |     yg = pR.primiRightside(j,end);
    |     x1 = exp(-ax/tScale*t1);
    |     des_c1 = linspace(0,max(t1),N_bf);    % point in time where to put the activation function
    |     c1 = exp(-ax/tScale*des_c1);             % point in x where to put the activation function
    |     h1 = N_bf^1.5*ones(1,N_bf)./c1;       % variance of each activation function, trial and error
    | 
    |     psi1 = zeros(N_bf,length(x1));
    |         for k = 1:N_bf
    |             for l = 1:length(x1)
    |                 psi1(k,l) = exp(-h1(k)*(x1(l)-c1(k))^2);
    |             end
    |         end    
    |         
    |     % Forcing term
    |     wpsi1 = w.wRightside(j,:)*psi1;
    |     f1 = wpsi1./(sum(psi1)).*x1*(yg-y0);
    |     
    |     % Reproducing
    |     ddyIm = zeros(1,length(t1));
    |     dyIm = zeros(1,length(t1));
    |     yIm = zeros(1,length(t1));
    |     
    |     if count == 1
    |         yIm(1) = pEnd.primiEndstep(j,end);
    |     else
    |         yIm(1) = pL.primiLeftside(j,end);
    |     end
    | 
    |     
    |     
    |     for k = 2:length(t1)
    |         ddyIm(k-1) = 1/tScale^2*(ay*(by*(yg-yIm(k-1))-tScale*dyIm(k-1))+f1(k-1));
    |         dyIm(k) = dyIm(k-1)+ddyIm(k-1)*dt;
    |         yIm(k) = yIm(k-1)+dyIm(k-1)*dt;  
    |     end
    |     
    |     anglesIm1(j,:) = yIm;
    | end
    | 
    | hPl = anglesIm1(1,:);
    | hPr = anglesIm1(2,:);
    | kBl = anglesIm1(3,:);
    | kBr = anglesIm1(4,:);
    | aPl = -hPl+kBl;%anglesIm1(5,:);
    | aPr = -hPr+kBr;%anglesIm1(6,:);
    | hRl = -anglesIm1(7,:);
    | hRr = -anglesIm1(8,:);
    | aRl = -anglesIm1(9,:);
    | aRr = -anglesIm1(10,:);
    | hYl = zeros(1,size(anglesIm1,2));   
    | hYr = zeros(1,size(anglesIm1,2));
    | 
    | 
    | % hPl = [anglesIm1(1,:) anglesIm1(1,:)];
    | % hPr = [anglesIm1(2,:) anglesIm1(2,:)];
    | % kBl = [anglesIm1(3,:) anglesIm1(3,:)];
    | % kBr = [anglesIm1(4,:) anglesIm1(4,:)];
    | % aPl = -hPl+kBl;%anglesIm1(5,:);
    | % aPr = -hPr+kBr;%anglesIm1(6,:);
    | % hRl = [-anglesIm1(7,:) anglesIm1(7,:)];
    | % hRr = [-anglesIm1(8,:) anglesIm1(8,:)];
    | % aRl = [-anglesIm1(9,:) anglesIm1(9,:)];
    | % aRr = [-anglesIm1(10,:) anglesIm1(10,:)];
    | % hYl = [zeros(1,size(anglesIm1,2)) zeros(1,size(anglesIm1,2))];   
    | % hYr = [zeros(1,size(anglesIm1,2)) zeros(1,size(anglesIm1,2))];
  function [hPl,hPr,kBl,kBr,aPl,aPr,hRl,hRr,aRl,aRr,hYl,hYr] = motionSideLeft(tScale,count):
    | function [hPl,hPr,kBl,kBr,aPl,aPr,hRl,hRr,aRl,aRr,hYl,hYr] = motionSideLeft(tScale,count)
    | 
    | 
    | w = load ('wLeftside.mat');
    | pEnd = load ('primiEndstep.mat');
    | pL = load ('primiLeftside.mat');
    | pR = load ('primiRightside.mat');
    | 
    | dt = 0.01;
    | N_dmp = 10;     % number of dmps, number of curves to be imitated 
    | N_bf = 50;     % number of basic activation function
    | weights = zeros(N_dmp,N_bf);
    | ay = 25;        % ay & by: constants of the second order system
    | by = ay/4;
    | t = 0:dt:dt*(size(pL.primiLeftside,2)-1);
    | t1 = 0:dt:tScale*t(end);
    | anglesIm1 = zeros(10,length(t1));
    | ax = 1;
    | %%
    | for j = 1:N_dmp
    |     
    |     y0 = pL.primiLeftside(j,1);
    |     yg = pL.primiLeftside(j,end);
    |     x1 = exp(-ax/tScale*t1);
    |     des_c1 = linspace(0,max(t1),N_bf);    % point in time where to put the activation function
    |     c1 = exp(-ax/tScale*des_c1);             % point in x where to put the activation function
    |     h1 = N_bf^1.5*ones(1,N_bf)./c1;       % variance of each activation function, trial and error
    | 
    |     psi1 = zeros(N_bf,length(x1));
    |         for k = 1:N_bf
    |             for l = 1:length(x1)
    |                 psi1(k,l) = exp(-h1(k)*(x1(l)-c1(k))^2);
    |             end
    |         end    
    |         
    |     % Forcing term
    |     wpsi1 = w.wLeftside(j,:)*psi1;
    |     f1 = wpsi1./(sum(psi1)).*x1*(yg-y0);
    |     
    |     % Reproducing
    |     ddyIm = zeros(1,length(t1));
    |     dyIm = zeros(1,length(t1));
    |     yIm = zeros(1,length(t1));
    |     
    | %     if count == 1
    | %         yIm(1) = pEnd.primiBegstep(j,end);
    | %     else
    |         yIm(1) = pR.primiRightside(j,end);
    | %     end
    | 
    |     
    |     
    |     for k = 2:length(t1)
    |         ddyIm(k-1) = 1/tScale^2*(ay*(by*(yg-yIm(k-1))-tScale*dyIm(k-1))+f1(k-1));
    |         dyIm(k) = dyIm(k-1)+ddyIm(k-1)*dt;
    |         yIm(k) = yIm(k-1)+dyIm(k-1)*dt;  
    |     end
    |     
    |     anglesIm1(j,:) = yIm;
    | end
    | 
    | 
    | hPl = anglesIm1(1,:);
    | hPr = anglesIm1(2,:);
    | kBl = anglesIm1(3,:);
    | kBr = anglesIm1(4,:);
    | aPl = -hPl+kBl;%anglesIm1(5,:);
    | aPr = -hPr+kBr;%anglesIm1(6,:);
    | hRl = -anglesIm1(7,:);
    | hRr = -anglesIm1(8,:);
    | aRl = -anglesIm1(9,:);
    | aRr = -anglesIm1(10,:);
    | hYl = zeros(1,size(anglesIm1,2));   
    | hYr = zeros(1,size(anglesIm1,2));
    | 
    | % hPl = [anglesIm1(1,:) anglesIm1(1,:)];
    | % hPr = [anglesIm1(2,:) anglesIm1(2,:)];
    | % kBl = [anglesIm1(3,:) anglesIm1(3,:)];
    | % kBr = [anglesIm1(4,:) anglesIm1(4,:)];
    | % aPl = -hPl+kBl;%anglesIm1(5,:);
    | % aPr = -hPr+kBr;%anglesIm1(6,:);
    | % hRl = [-anglesIm1(7,:) anglesIm1(7,:)];
    | % hRr = [-anglesIm1(8,:) anglesIm1(8,:)];
    | % aRl = [-anglesIm1(9,:) anglesIm1(9,:)];
    | % aRr = [-anglesIm1(10,:) anglesIm1(10,:)];
    | % hYl = [zeros(1,size(anglesIm1,2)) zeros(1,size(anglesIm1,2))];   
    | % hYr = [zeros(1,size(anglesIm1,2)) zeros(1,size(anglesIm1,2))];
  function [hPl,hPr,kBl,kBr,aPl,aPr,hRl,hRr,aRl,aRr,hYl,hYr] = motionKick(tScale):
    | function [hPl,hPr,kBl,kBr,aPl,aPr,hRl,hRr,aRl,aRr,hYl,hYr] = motionKick(tScale)
    | 
    | 
    | w = load ('wKicking.mat');
    | pK = load ('primiKicking.mat');
    | pL = load ('primiLeftside.mat');
    | pR = load ('primiRightside.mat');
    | 
    | dt = 0.01;
    | N_dmp = 10;     % number of dmps, number of curves to be imitated 
    | N_bf = 50;     % number of basic activation function
    | weights = zeros(N_dmp,N_bf);
    | ay = 25;        % ay & by: constants of the second order system
    | by = ay/4;
    | t = 0:dt:dt*(size(pK.primiKicking,2)-1);
    | t1 = 0:dt:tScale*t(end);
    | anglesIm1 = zeros(10,length(t1));
    | ax = 1;
    | %%
    | for j = 1:N_dmp
    |     
    |     y0 = pK.primiKicking(j,1);
    |     yg = pK.primiKicking(j,end);
    |     x1 = exp(-ax/tScale*t1);
    |     des_c1 = linspace(0,max(t1),N_bf);    % point in time where to put the activation function
    |     c1 = exp(-ax/tScale*des_c1);             % point in x where to put the activation function
    |     h1 = N_bf^1.5*ones(1,N_bf)./c1;       % variance of each activation function, trial and error
    | 
    |     psi1 = zeros(N_bf,length(x1));
    |         for k = 1:N_bf
    |             for l = 1:length(x1)
    |                 psi1(k,l) = exp(-h1(k)*(x1(l)-c1(k))^2);
    |             end
    |         end    
    |         
    |     % Forcing term
    |     wpsi1 = w.wKicking(j,:)*psi1;
    |     f1 = wpsi1./(sum(psi1)).*x1*(yg-y0);
    |     
    |     % Reproducing
    |     ddyIm = zeros(1,length(t1));
    |     dyIm = zeros(1,length(t1));
    |     yIm = zeros(1,length(t1));
    |     
    | %     if count == 1
    | %         yIm(1) = pEnd.primiBegstep(j,end);
    | %     else
    | %         yIm(1) = pL.primiLeftside(j,end);
    | %     end
    | 
    |     
    |     
    |     for k = 2:length(t1)
    |         ddyIm(k-1) = 1/tScale^2*(ay*(by*(yg-yIm(k-1))-tScale*dyIm(k-1))+f1(k-1));
    |         dyIm(k) = dyIm(k-1)+ddyIm(k-1)*dt;
    |         yIm(k) = yIm(k-1)+dyIm(k-1)*dt;  
    |     end
    |     
    |     anglesIm1(j,:) = yIm;
    | end
    | 
    | 
    | hPl = anglesIm1(1,:);
    | hPr = anglesIm1(2,:);
    | kBl = anglesIm1(3,:);
    | kBr = anglesIm1(4,:);
    | aPl = -hPl+kBl;%anglesIm1(5,:);
    | aPr = -hPr+kBr;%anglesIm1(6,:);
    | hRl = -anglesIm1(7,:);
    | hRr = -anglesIm1(8,:);
    | aRl = -anglesIm1(9,:);
    | aRr = -anglesIm1(10,:);
    | hYl = zeros(1,size(anglesIm1,2));   
    | hYr = zeros(1,size(anglesIm1,2));
